simulink model "kalman_static_sim"  (R2024a)
settings: Solver=ode23tb  StartTime=0.0  StopTime=20  RelTol=1e-3
values from neighbouring files (symbols this model uses):
  A = [[0 1]; [0 0]]    [kalman_static_ini.m]
  Ae = [[A, B]; [0, 0, 0]]    [kalman_static_ini.m]
  B = [0; 3/5*g]    [kalman_static_ini.m]
  Be = [B; 0]    [kalman_static_ini.m]
  C = [1 0]    [kalman_static_ini.m]
  Ce = [C, 0]    [kalman_static_ini.m]
  H = lqr(A.', C.', Q, R).'    [kalman_static_ini.m]
  He = lqr(Ae.', Ce.', Qe, Re).'    [kalman_static_ini.m]
  nd = Tt / Ts    (= 16)    [kalman_static_ini.m]
  Ts = 1e-3    (= 0.001)    [kalman_static_ini.m]
libraries: cstblocks x1
settings Model: Creator=miche  LastModifiedBy=pichim

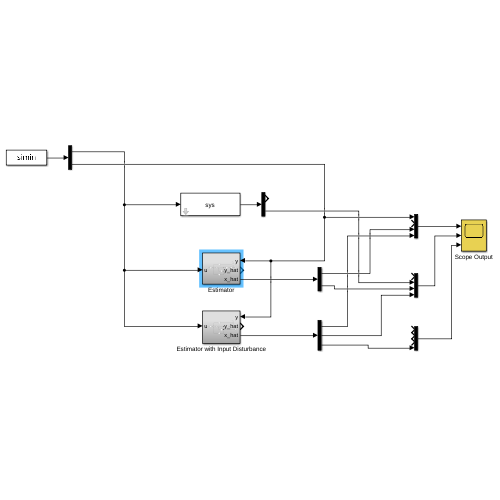
[thumbnail: Simulink's stored preview of the top-level diagram]
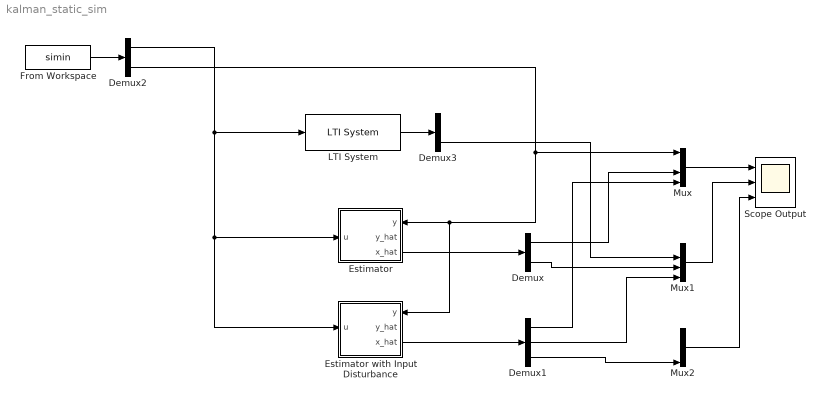
== system kalman_static_sim ==
  Demux : Demux  Outputs=2
  Demux1 : Demux  Outputs=3
  Demux2 : Demux  Outputs=2
  Demux3 : Demux  Outputs=2
  Estimator : Subsystem
      settings: PortSchema="{\"entries\":[{\"content\":{\"sides\":[{\"content\":{\"connectorIds\":[\"In1\"]},\"type\":\"ConnectorPlacement.EquallySpacedRectSide\",\"uuid\":\"2ab08da3-847e-4b02-ad4a-2ebe77e9daf7\"},{\"content\":{\"connectorIds\":[\"In2\",\"Out1\",\"Out2\"],\"side\":\"RIGHT\"},\"type\":\"ConnectorPlacement.EquallySpacedRectSide\",\"uuid\":\"e41fcd85-62bd-46ca-9c1a-184b8442f93d\"},{\"content\":{\"side\":\"TOP\"},\"type\":\"ConnectorPlacement.EquallySpacedRectSide\",\"uuid\":\"e71fc7b0-9d26-4f76-83b8-d38f8ea1d6de\"}]},\"type\":\"ConnectorPlacement.EquallySpacedConnector\",\"uuid\":\"ee2f8453-6783-49eb-a9ef-e927a515d773\"}],\"packageUris\":[\"http://schema.mathworks.com/mf0/Connector/R2020b\"],\"version\":\"1.0\"}"
  Estimator with Input Disturbance : Subsystem
      settings: PortSchema="{\"entries\":[{\"content\":{\"sides\":[{\"content\":{\"connectorIds\":[\"In1\"]},\"type\":\"ConnectorPlacement.EquallySpacedRectSide\",\"uuid\":\"2ab08da3-847e-4b02-ad4a-2ebe77e9daf7\"},{\"content\":{\"connectorIds\":[\"In2\",\"Out1\",\"Out2\"],\"side\":\"RIGHT\"},\"type\":\"ConnectorPlacement.EquallySpacedRectSide\",\"uuid\":\"e41fcd85-62bd-46ca-9c1a-184b8442f93d\"},{\"content\":{\"side\":\"TOP\"},\"type\":\"ConnectorPlacement.EquallySpacedRectSide\",\"uuid\":\"e71fc7b0-9d26-4f76-83b8-d38f8ea1d6de\"}]},\"type\":\"ConnectorPlacement.EquallySpacedConnector\",\"uuid\":\"ee2f8453-6783-49eb-a9ef-e927a515d773\"}],\"packageUris\":[\"http://schema.mathworks.com/mf0/Connector/R2020b\"],\"version\":\"1.0\"}"
  From Workspace : FromWorkspace  VariableName=simin  SampleTime=Ts
  LTI System : cstblocks/LTI System  sys=sys  IC=[]  PadeOrder=0
  Mux : Mux
  Mux1 : Mux
  Mux2 : Mux
  Scope Output : Scope  NumInputPorts=3
  wires:
  Demux2/2 -> Mux/1, Estimator with Input Disturbance/2(y), Estimator/2(y)
  Estimator/2(x_hat) -> Demux/1
  Mux/1 -> Scope Output/1
  Mux1/1 -> Scope Output/2
  Estimator with Input Disturbance/2(x_hat) -> Demux1/1
  Mux2/1 -> Scope Output/3
  Demux2/1 -> LTI System/1, Estimator with Input Disturbance/1(u), Estimator/1(u)
  From Workspace/1 -> Demux2/1
  LTI System/1 -> Demux3/1
  Demux/1 -> Mux/3
  Demux1/1 -> Mux/4
  Demux3/2 -> Mux1/2
  Demux/2 -> Mux1/3
  Demux1/2 -> Mux1/4
  Demux1/3 -> Mux2/4

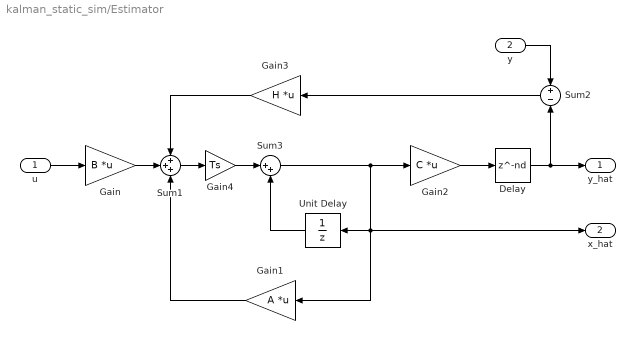
== system kalman_static_sim/Estimator ==
  u : Inport
  y : Inport  Port=2
  Delay : Delay  DelayLength=nd  SampleTime=Ts
  Gain : Gain  Gain=B  Multiplication=Matrix(K*u)
  Gain1 : Gain  Gain=A  Multiplication=Matrix(K*u)
  Gain2 : Gain  Gain=C  Multiplication=Matrix(K*u)
  Gain3 : Gain  Gain=H  Multiplication=Matrix(K*u)
  Gain4 : Gain  Gain=Ts
  Sum1 : Sum  Inputs=+++
  Sum2 : Sum  Inputs=+|-
  Sum3 : Sum  Inputs=|++
  Unit Delay : UnitDelay  SampleTime=Ts  HasFrameUpgradeWarning=on
  y_hat : Outport
  x_hat : Outport  Port=2
  wires:
  Unit Delay/1 -> Sum3/2
  Gain2/1 -> Delay/1
  Gain4/1 -> Sum3/1
  Sum3/1 -> Gain2/1, Gain1/1, x_hat/1, Unit Delay/1
  y/1 -> Sum2/1
  Delay/1 -> Sum2/2, y_hat/1
  u/1 -> Gain/1
  Sum1/1 -> Gain4/1
  Gain3/1 -> Sum1/1
  Sum2/1 -> Gain3/1
  Gain1/1 -> Sum1/3
  Gain/1 -> Sum1/2

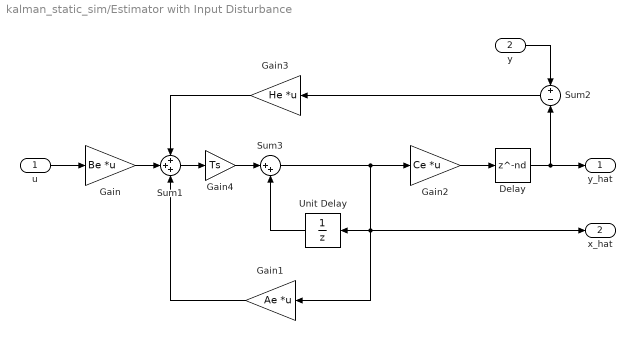
== system kalman_static_sim/Estimator with Input Disturbance ==
  u : Inport
  y : Inport  Port=2
  Delay : Delay  DelayLength=nd  SampleTime=Ts
  Gain : Gain  Gain=Be  Multiplication=Matrix(K*u)
  Gain1 : Gain  Gain=Ae  Multiplication=Matrix(K*u)
  Gain2 : Gain  Gain=Ce  Multiplication=Matrix(K*u)
  Gain3 : Gain  Gain=He  Multiplication=Matrix(K*u)
  Gain4 : Gain  Gain=Ts
  Sum1 : Sum  Inputs=+++
  Sum2 : Sum  Inputs=+|-
  Sum3 : Sum  Inputs=|++
  Unit Delay : UnitDelay  SampleTime=Ts  HasFrameUpgradeWarning=on
  y_hat : Outport
  x_hat : Outport  Port=2
  wires:
  Sum1/1 -> Gain4/1
  Delay/1 -> Sum2/2, y_hat/1
  y/1 -> Sum2/1
  Unit Delay/1 -> Sum3/2
  Sum3/1 -> Gain2/1, Gain1/1, x_hat/1, Unit Delay/1
  Gain4/1 -> Sum3/1
  Gain/1 -> Sum1/2
  Gain3/1 -> Sum1/1
  u/1 -> Gain/1
  Gain1/1 -> Sum1/3
  Gain2/1 -> Delay/1
  Sum2/1 -> Gain3/1
